simulink model "feedforeward"  (R2024b)
settings: Solver=VariableStepAuto  StartTime=0.0  StopTime=10  RelTol=1e-3
undefined symbols (not defined in the file or in its folder): ia_limite, kamp, kdt, kff, ki, klim, kp, kt, kv, S_new2, Vctr, Vnom
libraries: cstblocks x2, simulink x1
settings Model: Creator=turco  LastModifiedBy=turco

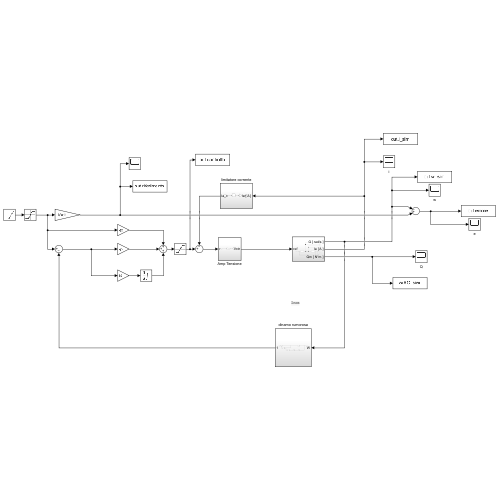
[thumbnail: Simulink's stored preview of the top-level diagram]
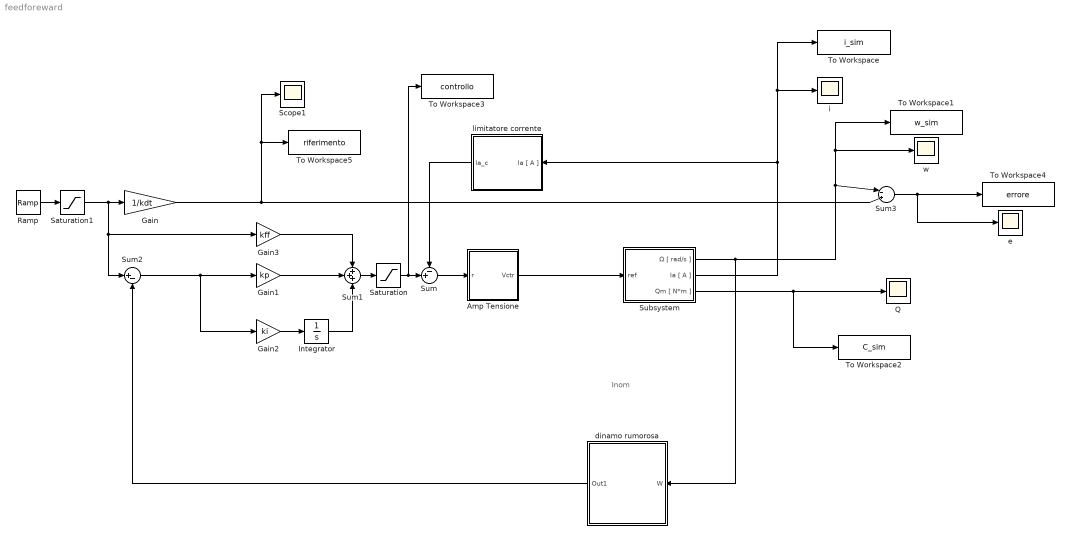
== system feedforeward ==
  note: Inom
  Amp Tensione : Subsystem
  Gain : Gain  Gain=1/kdt
  Gain1 : Gain  Gain=kp
  Gain2 : Gain  Gain=ki
  Gain3 : Gain  Gain=kff
  Integrator : Integrator  LimitOutput=on  UpperSaturationLimit=S_new2  LowerSaturationLimit=-S_new2
  Q : Scope
  Ramp : simulink/Sources/Ramp  slope=1  start=0  InitialOutput=0
  Saturation : Saturate  UpperLimit=5  LowerLimit=-5
  Saturation1 : Saturate  UpperLimit=Vctr*0.9  LowerLimit=-Vctr*0.9
  Scope1 : Scope
  Subsystem : Subsystem
  Sum : Sum  Inputs=-+|
  Sum1 : Sum  Inputs=+++
  Sum2 : Sum  Inputs=|+-
  Sum3 : Sum  Inputs=|-+|
  To Workspace : ToWorkspace  VariableName=i_sim  SaveFormat=Timeseries  SampleTime=-1
  To Workspace1 : ToWorkspace  VariableName=w_sim  SaveFormat=Timeseries  SampleTime=-1
  To Workspace2 : ToWorkspace  VariableName=C_sim  SaveFormat=Timeseries  SampleTime=-1
  To Workspace3 : ToWorkspace  VariableName=controllo  SaveFormat=Timeseries  SampleTime=-1
  To Workspace4 : ToWorkspace  VariableName=errore  SaveFormat=Timeseries  SampleTime=-1
  To Workspace5 : ToWorkspace  VariableName=riferimento  SaveFormat=Timeseries  SampleTime=-1
  dinamo rumorosa : Subsystem
  e : Scope
  i : Scope
  limitatore corrente : Subsystem
  w : Scope
  wires:
  Gain2/1 -> Integrator/1
  Subsystem/3(Qm [ N*m ]) -> To Workspace2/1, Q/1
  Sum2/1 -> Gain2/1, Gain1/1
  Subsystem/1(Ω [ rad/s ]) -> To Workspace1/1, w/1, Sum3/1, dinamo rumorosa/1(W)
  dinamo rumorosa/1(Out1) -> Sum2/2
  limitatore corrente/1(Ia_c) -> Sum/1
  Amp Tensione/1(Vctr) -> Subsystem/1(ref)
  Saturation/1 -> To Workspace3/1, Sum/2
  Subsystem/2(Ia [ A ]) -> To Workspace/1, i/1, limitatore corrente/1(Ia [ A ])
  Sum1/1 -> Saturation/1
  Sum/1 -> Amp Tensione/1(r)
  Gain/1 -> Sum3/2, Scope1/1, To Workspace5/1
  Sum3/1 -> e/1, To Workspace4/1
  Gain1/1 -> Sum1/2
  Integrator/1 -> Sum1/3
  Gain3/1 -> Sum1/1
  Ramp/1 -> Saturation1/1
  Saturation1/1 -> Gain3/1, Sum2/1, Gain/1

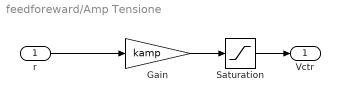
== system feedforeward/Amp Tensione ==
  r : Inport
  Gain : Gain  Gain=kamp
  Saturation : Saturate  UpperLimit=+Vnom*1.2  LowerLimit=-Vnom*1.2
  Vctr : Outport
  wires:
  r/1 -> Gain/1
  Saturation/1 -> Vctr/1
  Gain/1 -> Saturation/1

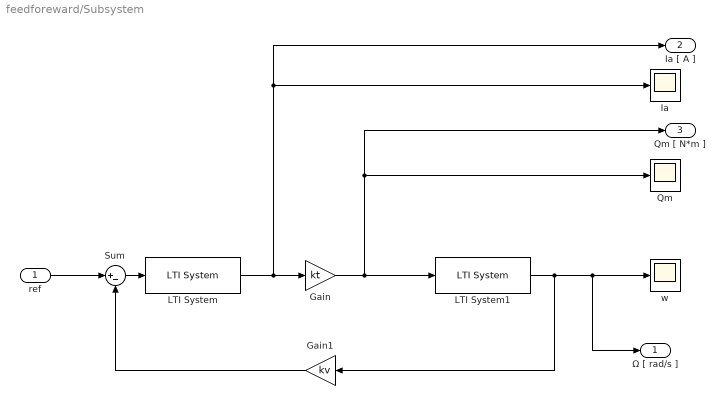
== system feedforeward/Subsystem ==
  ref : Inport
  Gain : Gain  Gain=kt
  Gain1 : Gain  Gain=kv
  Ia : Scope
  LTI System : cstblocks/LTI System  sys=Pel  IC=[]  PadeOrder=0
  LTI System1 : cstblocks/LTI System  sys=Pmec  IC=[]  PadeOrder=0
  "Qm " : Scope
  Sum : Sum  Inputs=|+-
  w : Scope
  Ω [ rad/s ] : Outport
  Ia [ A ] : Outport  Port=2
  Qm [ N*m ] : Outport  Port=3
  wires:
  LTI System1/1 -> Ω [ rad/s ]/1, w/1, Gain1/1
  Gain1/1 -> Sum/2
  Gain/1 -> Qm [ N*m ]/1, "Qm "/1, LTI System1/1
  Sum/1 -> LTI System/1
  LTI System/1 -> Ia [ A ]/1, Ia/1, Gain/1
  ref/1 -> Sum/1

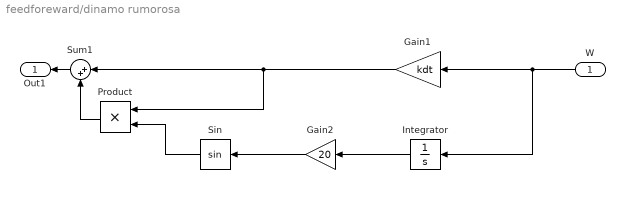
== system feedforeward/dinamo rumorosa ==
  W : Inport
  Gain1 : Gain  Gain=kdt
  Gain2 : Gain  Gain=20
  Integrator : Integrator
  Product : Product
  Sin : Trigonometry
  Sum1 : Sum  Inputs=|++
  Out1 : Outport
  wires:
  Integrator/1 -> Gain2/1
  Gain2/1 -> Sin/1
  W/1 -> Gain1/1, Integrator/1
  Product/1 -> Sum1/2
  Gain1/1 -> Product/1, Sum1/1
  Sin/1 -> Product/2
  Sum1/1 -> Out1/1

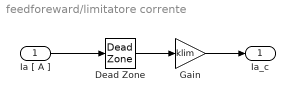
== system feedforeward/limitatore corrente ==
  Ia [ A ] : Inport
  Dead Zone : DeadZone  LowerValue=-ia_limite  UpperValue=+ia_limite
  Gain : Gain  Gain=klim
  Ia_c : Outport
  wires:
  Gain/1 -> Ia_c/1
  Ia [ A ]/1 -> Dead Zone/1
  Dead Zone/1 -> Gain/1
